simulink model "States5_2018a"  (R2018a)
settings: Solver=FixedStepDiscrete  StartTime=0.0  StopTime=1.0  FixedStep=0.1  RelTol=1e-3  EnableMultiTasking=on
settings Model: Creator=bzhan  LastModifiedBy=bzhan
settings SolverCC: AutoInsertRateTranBlk=on
settings DataIOCC: LimitDataPoints=on  ReturnWorkspaceOutputs=on
settings OptimizationCC: LifeSpan=inf
settings DebuggingCC: AllowSymbolicDim=off  SFUnexpectedBacktrackingDiag=warning  SFNoUnconditionalDefaultTransitionDiag=warning  SFExecutionAtInitializationDiag=none
settings CodeAppCC: StateflowObjectComments=on
settings GRTTargetCC: TargetLangStandard=C89/C90 (ANSI)
settings ConfigComp: CovMetricSettings=dw  CovHtmlReporting=on  CovSaveCumulativeToWorkspaceVar=on  CovSaveSingleToWorkspaceVar=on  CovShowResultsExplorer=off  CovExternalEMLEnable=off  CovSFcnEnable=off

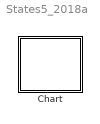
== system States5_2018a ==
  Chart : Stateflow chart  TreatAsAtomicUnit=on

== stateflow chart States5_2018a/Chart ==
  settings: updateMethod=DISCRETE  sampleTime=0.1
  state A
    (history)
    state A2
      en: f("enA2")
    state A1
      en: f("enA1")
    (default) -> A1
    A1 -> A2 : {x=x+1;}
    A2 -> A1 : {x=x+1;}
  state B
    state B2
      en: f("enB2")
    state B1
      en: f("enB1")
    (default) -> B1
    B1 -> B2 : {x=x-1;}
    B2 -> B1 : {x=x-1;}
  (default) -> A : {x=0;}
  A -> B : [x>=1]
  B -> A : [x<=0]
  data: s function_input; x local
  function f(s):
    | function f(s)
    |   fprintf(s+"\n");
